simulink model "symulink"  (R2017a)
settings: Solver=VariableStepAuto  StartTime=0.0  StopTime=100  RelTol=1e-3
values from neighbouring files (symbols this model uses):
  A = [0 0 1 0]    [Linearyzacja_ramienia_robota.m]    (also in model_nie_liniowy.m = [0 0 1 0; sciaga.m; zad1.m = double(A); zad1_v3.m = double(A))
  B = [0 0; 0 0; double(d1); double(d2)]    [Linearyzacja_ramienia_robota.m]    (also in model_nie_liniowy.m = [0 0; sciaga.m; zad1.m = [0 0; zad1_v3.m = [0 0)
  C = [1 0 0 0; 0 1 0 0]    [Linearyzacja_ramienia_robota.m]    (also in model_nie_liniowy.m = [1 0 0 0; sciaga.m = [1 0 0 0; 0 1 0 0; 0 0 1 0; 0 0 0 1]; zad1.m = eye(4); zad1_od_nowa.m = eye(4))
  KFeedBack = place(A,B,[-15,-6,-9,-12])    [zad1.m]    (also in zad1_v3.m = place(A,B,[-1,-3,-5,-7]))
settings Model: Creator=Szwank  LastModifiedBy=Szwank

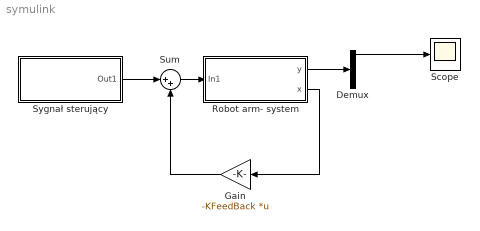
== system symulink ==
  Demux : Demux
  Gain : Gain  Gain=-KFeedBack  Multiplication=Matrix(K*u)
  Robot arm- system : Subsystem
  Scope : Scope
  Sum : Sum  Inputs=|++
  Sygnał sterujący : Subsystem
  wires:
  Robot arm- system/2(x) -> Gain/1
  Gain/1 -> Sum/2
  Sum/1 -> Robot arm- system/1(In1)
  Robot arm- system/1(y) -> Demux/1
  Sygnał sterujący/1(Out1) -> Sum/1
  Demux/1 -> Scope/1

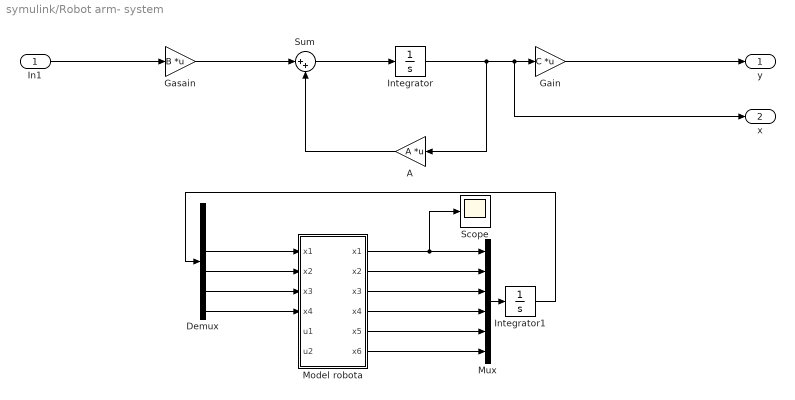
== system symulink/Robot arm- system ==
  In1 : Inport
  A : Gain  Gain=A  Multiplication=Matrix(K*u)
  Demux : Demux  Outputs=6
  Gain : Gain  Gain=C  Multiplication=Matrix(K*u)
  Gasain : Gain  Gain=B  Multiplication=Matrix(K*u)
  Integrator : Integrator  InitialCondition=[0 0 0 0]
  Integrator1 : Integrator
  Model robota : MATLAB Function  TreatAsAtomicUnit=on
  Mux : Mux  Inputs=6
  Scope : Scope
  Sum : Sum  Inputs=|++
  y : Outport
  x : Outport  Port=2
  wires:
  In1/1 -> Gasain/1
  Gasain/1 -> Sum/1
  A/1 -> Sum/2
  Sum/1 -> Integrator/1
  Integrator/1 -> x/1, Gain/1, A/1
  Gain/1 -> y/1
  Model robota/1(x1) -> Scope/1, Mux/1
  Model robota/2(x2) -> Mux/2
  Model robota/3(x3) -> Mux/3
  Model robota/4(x4) -> Mux/4
  Model robota/5(x5) -> Mux/5
  Model robota/6(x6) -> Mux/6
  Mux/1 -> Integrator1/1
  Integrator1/1 -> Demux/1
  Demux/6 -> Model robota/4("x4 ")
  Demux/5 -> Model robota/3("x3 ")
  Demux/4 -> Model robota/2("x2 ")
  Demux/3 -> Model robota/1("x1 ")

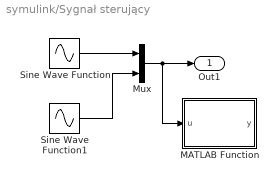
== system symulink/Sygnał sterujący ==
  MATLAB Function : MATLAB Function  TreatAsAtomicUnit=on
  Mux : Mux  Inputs=2
      settings: DisplayOption=signals
  Sine Wave Function : Sin  TimeSource=Use external signal  Amplitude=30  SampleTime=0
  Sine Wave Function1 : Sin  TimeSource=Use external signal  Phase=pi/2  SampleTime=0
  Out1 : Outport
  wires:
  Mux/1 -> MATLAB Function/1(u), Out1/1
  Sine Wave Function/1 -> Mux/1
  Sine Wave Function1/1 -> Mux/2

== matlab function symulink/Sygnał sterujący/MATLAB Function ==
  data: u input; y output
function y = fcn(u)

y = u;

== matlab function symulink/Robot arm- system/Model robota ==
  data: x1 output; x2 output; x3 output; x4 output; x1 input; x5 output; x2 input; x3 input; x4 input; u1 input; u2 input; x6 output
function [x1, x2, x3, x4, x5, x6] = fcn(x1, x2, x3, x4, u1, u2)

m1 = 2;
m2 = 1;
L1 = 1.5;
Lc1 = L1/2;
L2 = 1;
Lc2 = L2/2;
g = 9.81;

H11 = m1* Lc1^2 + J1 + m2 * (L1^2 + Lc2^2 + 2*L1*L2*cos(x2));
H22 = m1 * Lc1^2 +J2;
H12 = m2 * L1*L2*cos(x2) + m2*Lc2 + J2;
H21 = H12;
h = m2*L1*Lc2*sin(x2);
g1 = m1*Lc1*g*cos(x1) + m2*g*(Lc2*cos(x1+x2) + L1*cos(x1));
g2 = m2*Lc2*g*cos(x1+x2);

F1 = (H22*H11-H12*H21)/H22;
F2 = (-H11*H22 + H12*H21)/H21;

x6 = -H11*(T2 - h*x3^2 - g2)/(-H11*H22 + H12*H21) + h*x4*x3/F2 - ((-h*x3 - h*x4)*x4)/F2 - g1/F2 + T1/F2;
x5 = -H12*(T2 - h*x3^2 - g2)/(H22*H11 - H12*H21) + h*x4*x3/F1 - (-h*x1-h*x4)*x3/F1 - g/F1 + T1/F1;

y = u;
